simulink model "PulseSimulation"  (R2024b)
settings: Solver=VariableStepAuto  StartTime=0.0  StopTime=2e-3  RelTol=1e-3
settings Model: Creator=castl  LastModifiedBy=castl

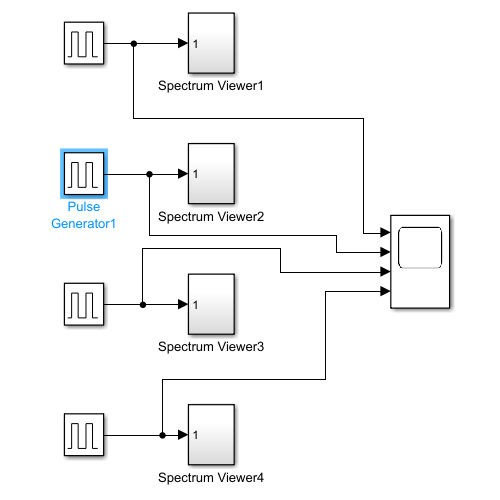
[thumbnail: Simulink's stored preview of the top-level diagram]
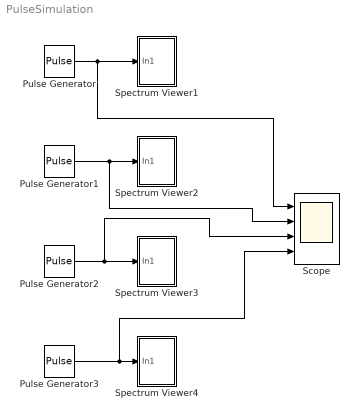
== system PulseSimulation ==
  Pulse Generator : DiscretePulseGenerator  PulseType=Time based  Period=5e-4  PulseWidth=2.5
  Pulse Generator1 : DiscretePulseGenerator  PulseType=Time based  Period=5e-4  PulseWidth=10
  Pulse Generator2 : DiscretePulseGenerator  PulseType=Time based  Period=2.5e-4  PulseWidth=10
  Pulse Generator3 : DiscretePulseGenerator  PulseType=Time based  Period=2.5e-4  PulseWidth=20
  Scope : Scope  NumInputPorts=4
  Spectrum Viewer1 : Subsystem
  Spectrum Viewer2 : Subsystem
  Spectrum Viewer3 : Subsystem
  Spectrum Viewer4 : Subsystem
  wires:
  Pulse Generator3/1 -> Scope/4, Spectrum Viewer4/1(In1)
  Pulse Generator2/1 -> Scope/3, Spectrum Viewer3/1(In1)
  Pulse Generator1/1 -> Scope/2, Spectrum Viewer2/1(In1)
  Pulse Generator/1 -> Scope/1, Spectrum Viewer1/1(In1)

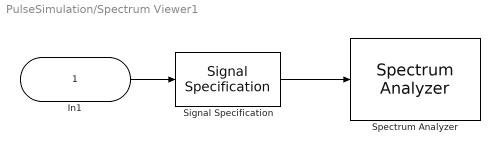
== system PulseSimulation/Spectrum Viewer1 ==
  In1 : Inport
  Signal Specification : SignalSpecification  SampleTime=1/16e4
  Spectrum Analyzer : SpectrumAnalyzer  WindowPosition=[775.000000,284.000000,800.000000,782.000000,]  ScopeFrameLocation=window  Method=Welch  AxesScaling=Manual  FrequencyResolutionMethod=Window length  FrequencySpan=Span and center frequency  Span=160000  StartFrequency=-80000  StopFrequency=80000  OverlapPercent=6.25  AveragingMethod=Running  SpectralAverages=200  SpectrumUnits=Watts  YLimits=[-0.0005915512961026187,0.0015937440463543971]  AllowFFTLengthLessThanSamplesPerUpdate=on  DefaultConfigurationName=spbscopes.SpectrumAnalyzerBlockCfg  IsFrequencyInputMode=0  FrequencyVectorPort=0  FrequencyVectorFromPort=0  FrequencyInputRBWPort=0  FrequencyInputRBWFromPort=0
  wires:
  In1/1 -> Signal Specification/1
  Signal Specification/1 -> Spectrum Analyzer/1

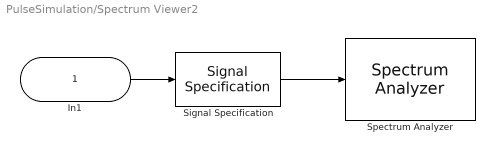
== system PulseSimulation/Spectrum Viewer2 ==
  In1 : Inport
  Signal Specification : SignalSpecification  SampleTime=1/16e4
  Spectrum Analyzer : SpectrumAnalyzer  WindowPosition=[182.000000,63.000000,800.000000,782.000000,]  ScopeFrameLocation=window  Method=Welch  AxesScaling=Manual  FrequencyResolutionMethod=Window length  FrequencySpan=Span and center frequency  Span=160000  StartFrequency=-80000  StopFrequency=80000  OverlapPercent=6.25  AveragingMethod=Running  SpectralAverages=200  SpectrumUnits=Watts  YLimits=[-0.002473110450553474,0.0024221627351022315]  SelectedToolstripTab=spectrumAnalyzerToolstrip.spectrumTab  AllowFFTLengthLessThanSamplesPerUpdate=on  DefaultConfigurationName=spbscopes.SpectrumAnalyzerBlockCfg  IsFrequencyInputMode=0  FrequencyVectorPort=0  FrequencyVectorFromPort=0  FrequencyInputRBWPort=0  FrequencyInputRBWFromPort=0
  wires:
  In1/1 -> Signal Specification/1
  Signal Specification/1 -> Spectrum Analyzer/1

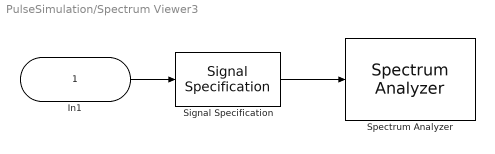
== system PulseSimulation/Spectrum Viewer3 ==
  In1 : Inport
  Signal Specification : SignalSpecification  SampleTime=1/16e4
  Spectrum Analyzer : SpectrumAnalyzer  WindowPosition=[16.000000,437.000000,800.000000,782.000000,]  ScopeFrameLocation=window  Method=Welch  AxesScaling=Manual  FrequencyResolutionMethod=Window length  FrequencySpan=Span and center frequency  Span=160000  StartFrequency=-80000  StopFrequency=80000  OverlapPercent=6.25  AveragingMethod=Running  SpectralAverages=200  SpectrumUnits=Watts  YLimits=[-0.003504166523373956,0.007181600916781373]  SelectedToolstripTab=spectrumAnalyzerToolstrip.spectrumTab  AllowFFTLengthLessThanSamplesPerUpdate=on  DefaultConfigurationName=spbscopes.SpectrumAnalyzerBlockCfg  IsFrequencyInputMode=0  FrequencyVectorPort=0  FrequencyVectorFromPort=0  FrequencyInputRBWPort=0  FrequencyInputRBWFromPort=0
  wires:
  In1/1 -> Signal Specification/1
  Signal Specification/1 -> Spectrum Analyzer/1

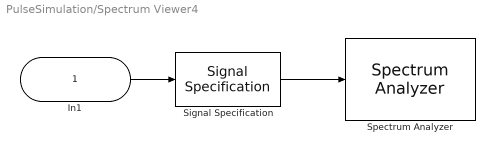
== system PulseSimulation/Spectrum Viewer4 ==
  In1 : Inport
  Signal Specification : SignalSpecification  SampleTime=1/16e4
  Spectrum Analyzer : SpectrumAnalyzer  WindowPosition=[1600.000000,284.000000,800.000000,782.000000,]  ScopeFrameLocation=window  Method=Welch  AxesScaling=Manual  FrequencyResolutionMethod=Window length  FrequencySpan=Span and center frequency  Span=160000  StartFrequency=-80000  StopFrequency=80000  OverlapPercent=6.25  AveragingMethod=Running  SpectralAverages=200  SpectrumUnits=Watts  YLimits=[-0.030316606322255156,0.06489473146714564]  SelectedToolstripTab=spectrumAnalyzerToolstrip.spectrumTab  AllowFFTLengthLessThanSamplesPerUpdate=on  DefaultConfigurationName=spbscopes.SpectrumAnalyzerBlockCfg  IsFrequencyInputMode=0  FrequencyVectorPort=0  FrequencyVectorFromPort=0  FrequencyInputRBWPort=0  FrequencyInputRBWFromPort=0
  wires:
  In1/1 -> Signal Specification/1
  Signal Specification/1 -> Spectrum Analyzer/1
